simulink model "Copy_of_Controller"  (R2018b)
settings: configuration reference "control_config" (kept outside this file)
values from neighbouring files (symbols this model uses):
  CONTROL_EXPORT = Simulink.Parameter(CONTROL_EXPORT_VALUE)    [controller_model_init.m]
  CONTROL_PARAM = Simulink.Parameter(CONTROL_PARAM_VALUE)    [controller_model_init.m]
undefined symbols (not defined in the file or in its folder): actuator_cmd, CONTROL_CONST, ControlMode, DiscIntNeverNeededParam, phi_cmd, theta_cmd, timestamp, w_cmd
libraries: simulink x34, FMT_Model_Lib x19
(part 1 of 4)
settings Model: Creator=jc  LastModifiedBy=zouji
settings ConfigSetRef: SourceLocation=Base Workspace

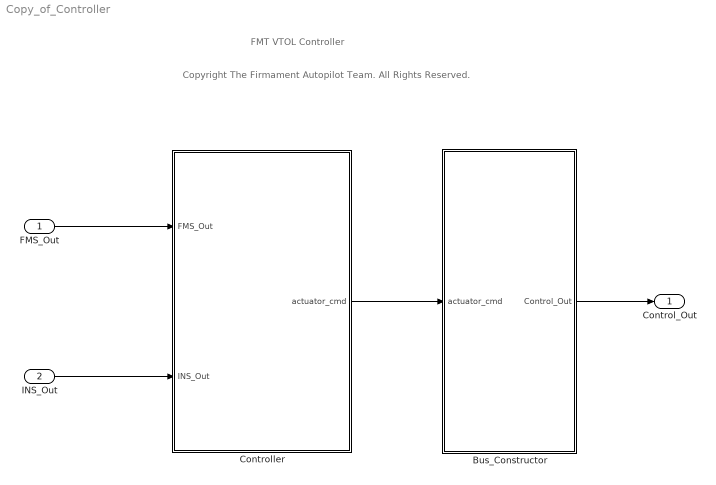
== system Copy_of_Controller ==
  note: Copyright The Firmament Autopilot Team. All Rights Reserved.
  note: FMT VTOL Controller
  FMS_Out : Inport  OutDataTypeStr=Bus: FMS_Out_Bus
  INS_Out : Inport  Port=2  OutDataTypeStr=Bus: INS_Out_Bus
  Bus_Constructor : Subsystem
  Controller : Subsystem
  Control_Out : Outport  OutDataTypeStr=Bus: Control_Out_Bus
  wires:
  FMS_Out/1 -> Controller/1(FMS_Out)
  INS_Out/1 -> Controller/2(INS_Out)
  Controller/1(actuator_cmd) -> Bus_Constructor/1(actuator_cmd)
  Bus_Constructor/1(Control_Out) -> Control_Out/1

== system Copy_of_Controller/Bus_Constructor ==
  actuator_cmd : Inport
  Bus Assignment : BusAssignment  AssignedSignals=actuator_cmd,timestamp
  Constant : Constant  Value=0  OutDataTypeStr=Bus: Control_Out_Bus
  timestamp : Subsystem  mask{sample_time=CONTROL_EXPORT.period}
      mask prompts: sample_time "sample time (ms)"
  Control_Out : Outport
  wires:
  actuator_cmd/1 -> Bus Assignment/2
  Constant/1 -> Bus Assignment/1
  Bus Assignment/1 -> Control_Out/1
  timestamp/1(timestamp_ms) -> Bus Assignment/3

== system Copy_of_Controller/Controller ==
  FMS_Out : Inport
  INS_Out : Inport  Port=2
  FW_Controller : Subsystem  TreatAsAtomicUnit=on
  MC_Controller : Subsystem  TreatAsAtomicUnit=on
  Merge : Merge
  VTOL_Control_Allocation : Subsystem
  switch-case : Subsystem
  actuator_cmd : Outport
  wires:
  INS_Out/1 -> MC_Controller/2(INS_Out), FW_Controller/2(INS_Out)
  FW_Controller/1(VTOL_actuator_cmd) -> Merge/1
  switch-case/1(FW_Trigger) -> FW_Controller/Action
  switch-case/2(MC_Trigger) -> MC_Controller/Action
  FMS_Out/1 -> MC_Controller/1(FMS_Out), FW_Controller/1(FMS_Out), VTOL_Control_Allocation/1(FMS_Out), switch-case/1(FMS_Out)
  MC_Controller/1(VTOL_actuator_cmd) -> Merge/2
  Merge/1 -> VTOL_Control_Allocation/2(VTOL_actuator_cmd)
  VTOL_Control_Allocation/1(actuator_cmd) -> actuator_cmd/1

== system Copy_of_Controller/Bus_Constructor/timestamp ==
  Constant : Constant  Value=sample_time
  Data Type Conversion : DataTypeConversion  OutDataTypeStr=uint32
  Discrete-Time Integrator : DiscreteIntegrator  IntegratorMethod=Accumulation: Forward Euler  SampleTime=-1  ICPrevOutput=DiscIntNeverNeededParam  ICPrevScaledInput=DiscIntNeverNeededParam
  timestamp_ms : Outport
  wires:
  Discrete-Time Integrator/1 -> Data Type Conversion/1
  Constant/1 -> Discrete-Time Integrator/1
  Data Type Conversion/1 -> timestamp_ms/1

== system Copy_of_Controller/Controller/FW_Controller ==
  FMS_Out : Inport
  INS_Out : Inport  Port=2
  Action Port : ActionPort  InitializeStates=reset  ActionType=case
  Aux_MC_Controller : Subsystem
  Effective_Factor : Subsystem
  FW_Controller : Subsystem
  Signal_Select : Subsystem
  VTOL_actuator_cmd : Outport  VectorParamsAs1DForOutWhenUnconnected=on
  wires:
  INS_Out/1 -> Aux_MC_Controller/3(INS_Out), FW_Controller/2(INS_Out), Effective_Factor/2(INS_Out)
  FW_Controller/3(aux_mc_cmd) -> Aux_MC_Controller/2(aux_cmd)
  FMS_Out/1 -> Aux_MC_Controller/1(FMS_Out), Signal_Select/1(FMS_Out), FW_Controller/1(FMS_Out), Effective_Factor/1(FMS_Out)
  Effective_Factor/2(factor_fw) -> FW_Controller/4(factor_fw)  "factor_fw"
  Effective_Factor/3(factor_mc) -> Aux_MC_Controller/4(factor_mc)  "factor_mc"
  Effective_Factor/1(VT) -> FW_Controller/3(VT)
  FW_Controller/1(fw_torque_cmd) -> Signal_Select/2(fw_torque_cmd)  "fw_torque_cmd"
  FW_Controller/2(fw_force_cmd) -> Signal_Select/3(fw_force_cmd)  "fw_force_cmd"
  Aux_MC_Controller/1(mc_torque_cmd) -> Signal_Select/4(mc_torque_cmd)  "aux_torque_cmd"
  Aux_MC_Controller/2(mc_force_cmd) -> Signal_Select/5(mc_force_cmd)  "aux_force_cmd"
  Signal_Select/1(VTOL_actuator_cmd) -> VTOL_actuator_cmd/1

== system Copy_of_Controller/Controller/MC_Controller ==
  FMS_Out : Inport
  INS_Out : Inport  Port=2
  Action Port : ActionPort  InitializeStates=reset  ActionType=default
  Bus Creator : BusCreator  Inputs=4
  Constant : Constant  Value=[0;0;0]  VectorParams1D=off  OutDataTypeStr=single
  Constant1 : Constant  Value=[0;0;0]  VectorParams1D=off  OutDataTypeStr=single
  Horizontal_Control : Subsystem
  Vertical_Control : Subsystem
  VTOL_actuator_cmd : Outport
  wires:
  Bus Creator/1 -> VTOL_actuator_cmd/1
  Horizontal_Control/1(torque_cmd_B) -> Bus Creator/3  "mc_torque_cmd"
  INS_Out/1 -> Vertical_Control/2(INS_Out), Horizontal_Control/2(INS_Out)
  Vertical_Control/1(force_cmd_B) -> Bus Creator/4  "mc_force_cmd"
  FMS_Out/1 -> Vertical_Control/1(FMS_Out), Horizontal_Control/1(FMS_Out)
  Constant/1 -> Bus Creator/1  "fw_torque_cmd"
  Constant1/1 -> Bus Creator/2  "fw_force_cmd"

== system Copy_of_Controller/Controller/VTOL_Control_Allocation ==
  FMS_Out : Inport
  VTOL_actuator_cmd : Inport  Port=2
  Bus Selector : BusSelector  OutputSignals=mc_torque_cmd,mc_force_cmd,fw_torque_cmd,fw_force_cmd
  Bus_Construct : Subsystem
  VTOL_Control_Allocation : Subsystem  Variant=on
      settings: GeneratePreprocessorConditionals=on
  actuator_cmd : Outport  VectorParamsAs1DForOutWhenUnconnected=on
  wires:
  FMS_Out/1 -> VTOL_Control_Allocation/1(FMS_Out)
  Bus_Construct/1(actuator_cmd) -> actuator_cmd/1
  VTOL_Control_Allocation/1(actuator_cmd) -> Bus_Construct/1(vtol_actuator_cmd)
  VTOL_actuator_cmd/1 -> Bus Selector/1
  Bus Selector/1 -> VTOL_Control_Allocation/2(mc_torque_cmd)  "<mc_torque_cmd>"
  Bus Selector/2 -> VTOL_Control_Allocation/3(mc_force_cmd)  "<mc_force_cmd>"
  Bus Selector/3 -> VTOL_Control_Allocation/4(fw_torque_cmd)  "<fw_torque_cmd>"
  Bus Selector/4 -> VTOL_Control_Allocation/5(fw_force_cmd)  "<fw_force_cmd>"

== system Copy_of_Controller/Controller/switch-case ==
  FMS_Out : Inport
  Bus Selector : BusSelector  OutputSignals=ext_state
  Data Type Conversion : DataTypeConversion  OutDataTypeStr=Enum: VTOLState
  Switch Case1 : SwitchCase  CaseConditions={[VTOLState.Fixwing, VTOLState.ForwardTrans, VTOLState.BackwardTrans, VTOLState.Stall]}
  FW_Trigger : Outport  VectorParamsAs1DForOutWhenUnconnected=on
  MC_Trigger : Outport  Port=2  VectorParamsAs1DForOutWhenUnconnected=on
  wires:
  Data Type Conversion/1 -> Switch Case1/1
  FMS_Out/1 -> Bus Selector/1
  Bus Selector/1 -> Data Type Conversion/1  "<ext_state>"
  Switch Case1/2 -> MC_Trigger/1
  Switch Case1/1 -> FW_Trigger/1

== system Copy_of_Controller/Controller/FW_Controller/Aux_MC_Controller ==
  FMS_Out : Inport
  aux_cmd : Inport  Port=2
  INS_Out : Inport  Port=3
  factor_mc : Inport  Port=4
  Attitude_Controller : Subsystem
  Aux_Commander : Subsystem
  Saturation1 : Saturate  UpperLimit=1  LowerLimit=-1
  Saturation2 : Saturate  UpperLimit=1  LowerLimit=-1
  Vertical_Control : Subsystem
  mc_torque_cmd : Outport
  mc_force_cmd : Outport  Port=2  VectorParamsAs1DForOutWhenUnconnected=on
  wires:
  INS_Out/1 -> Attitude_Controller/2(INS_Out), Vertical_Control/3(INS_Out)
  aux_cmd/1 -> Aux_Commander/1(aux_cmd)
  FMS_Out/1 -> Aux_Commander/2(FMS_Out)
  Aux_Commander/1(Aux_FMS_Out) -> Attitude_Controller/1(FMS_Out), Vertical_Control/2(FMS_Out)
  Attitude_Controller/1(rate_dot_cmd_B) -> Saturation2/1
  Saturation2/1 -> mc_torque_cmd/1
  Vertical_Control/1(force_cmd_B) -> Saturation1/1
  Saturation1/1 -> mc_force_cmd/1
  factor_mc/1 -> Vertical_Control/1(factor_mc), Attitude_Controller/3(factor_mc)

== system Copy_of_Controller/Controller/FW_Controller/Effective_Factor ==
  FMS_Out : Inport
  INS_Out : Inport  Port=2
  Bus Selector : BusSelector  OutputSignals=ext_state
  Constant : Constant  Value=0  OutDataTypeStr=single
  Constant1 : Constant  OutDataTypeStr=single
  Constant2 : Constant  OutDataTypeStr=single
  Constant6 : Constant  Value=0  OutDataTypeStr=single
  Demux : Demux  Outputs=2
  First Order LPF1 : FMT_Model_Lib/Filter/First Order LPF  fc=1
      settings: SourceProductName=FMT Toolbox
  First Order LPF3 : FMT_Model_Lib/Filter/First Order LPF  fc=0.5
      settings: SourceProductName=FMT Toolbox
  Fly_Speed : Subsystem
  Multiport Switch : MultiPortSwitch  DataPortOrder=Zero-based contiguous  Inputs=5  zeroidx=on
  Mux : Mux  Inputs=2
  Mux2 : Mux  Inputs=2
  VT : Outport  VectorParamsAs1DForOutWhenUnconnected=on
  factor_fw : Outport  Port=2  VectorParamsAs1DForOutWhenUnconnected=on
  factor_mc : Outport  Port=3  VectorParamsAs1DForOutWhenUnconnected=on
  wires:
  INS_Out/1 -> Fly_Speed/1(INS_Out)
  Fly_Speed/1(VT) -> VT/1  "VT"
  FMS_Out/1 -> Bus Selector/1
  Bus Selector/1 -> Multiport Switch/1  "<ext_state>"
  Constant/1 -> Mux/1
  Constant1/1 -> Mux/2
  First Order LPF1/1 -> factor_fw/1
  First Order LPF3/1 -> factor_mc/1
  Mux/1 -> Multiport Switch/2, Multiport Switch/3, Multiport Switch/5, Multiport Switch/6
  Mux2/1 -> Multiport Switch/4
  Constant2/1 -> Mux2/1
  Constant6/1 -> Mux2/2
  Multiport Switch/1 -> Demux/1
  Demux/2 -> First Order LPF3/1
  Demux/1 -> First Order LPF1/1

== system Copy_of_Controller/Controller/FW_Controller/FW_Controller ==
  FMS_Out : Inport
  INS_Out : Inport  Port=2
  VT : Inport  Port=3
  factor_fw : Inport  Port=4
  Attitude_Control : Subsystem
  Lateral_Control : Subsystem
  Mux : Mux  Inputs=2
  Saturation1 : Saturate  UpperLimit=1  LowerLimit=-1
  Selector : Selector  InputPortWidth=3  IndexOptions=Index vector (dialog)  Indices=1  OutputSizes=1
  TECS_Core : Subsystem
  Throttle_Command : Subsystem
  fw_torque_cmd : Outport  VectorParamsAs1DForOutWhenUnconnected=on
  fw_force_cmd : Outport  Port=2  VectorParamsAs1DForOutWhenUnconnected=on
  aux_mc_cmd : Outport  Port=3  VectorParamsAs1DForOutWhenUnconnected=on
  wires:
  INS_Out/1 -> TECS_Core/1(INS_Out), Lateral_Control/2(INS_Out), Attitude_Control/4(INS_Out)
  Lateral_Control/1(phi_cmd) -> Mux/1  "fw_phi_cmd"
  Mux/1 -> Attitude_Control/5(att_cmd)
  TECS_Core/1(theta_cmd) -> Mux/2  "fw_theta_cmd"
  FMS_Out/1 -> TECS_Core/2(FMS_Out), Throttle_Command/2(FMS_Out), Lateral_Control/1(FMS_Out), Attitude_Control/2(FMS_Out)
  Attitude_Control/1(ang_acc_cmd) -> Saturation1/1
  Saturation1/1 -> fw_torque_cmd/1
  VT/1 -> Attitude_Control/3(VT), TECS_Core/3(VT)
  Attitude_Control/2(aux_mc_cmd) -> Selector/1, aux_mc_cmd/1  "aux_mc_cmd"
  TECS_Core/2(throttle_cmd) -> Throttle_Command/1(fw_throttle_cmd)  "fw_throttle_cmd"
  Throttle_Command/1(fw_force_cmd) -> fw_force_cmd/1
  Selector/1 -> TECS_Core/4(fw_phi_sp)
  factor_fw/1 -> Attitude_Control/1(factor_fw)

== system Copy_of_Controller/Controller/FW_Controller/Signal_Select ==
  FMS_Out : Inport
  fw_torque_cmd : Inport  Port=2
  fw_force_cmd : Inport  Port=3
  mc_torque_cmd : Inport  Port=4
  mc_force_cmd : Inport  Port=5
  Bus Creator : BusCreator  Inputs=4
  Bus Selector1 : BusSelector  OutputSignals=ctrl_mode
  Manual : simulink/Logic and Bit Operations/Compare To Constant  relop===  const=uint8(ControlMode.Manual)  OutDataTypeStr=boolean
  Manual_Command : Subsystem
  Switch : Switch  Criteria=u2 > Threshold
  VTOL_actuator_cmd : Outport
  wires:
  mc_force_cmd/1 -> Bus Creator/4  "mc_force_cmd"
  fw_torque_cmd/1 -> Bus Creator/1  "fw_torque_cmd"
  fw_force_cmd/1 -> Bus Creator/2  "fw_force_cmd"
  mc_torque_cmd/1 -> Bus Creator/3  "mc_torque_cmd"
  Bus Selector1/1 -> Manual/1  "<ctrl_mode>"
  FMS_Out/1 -> Manual_Command/1(FMS_Out), Bus Selector1/1
  Manual/1 -> Switch/2
  Bus Creator/1 -> Switch/3
  Switch/1 -> VTOL_actuator_cmd/1
  Manual_Command/1(vtol_actuator_cmd) -> Switch/1

== system Copy_of_Controller/Controller/MC_Controller/Horizontal_Control ==
  FMS_Out : Inport
  INS_Out : Inport  Port=2
  Attitude_Controller : Subsystem
  Velocity_Controller : Subsystem
  torque_cmd_B : Outport
  wires:
  Attitude_Controller/1(rate_dot_cmd_B) -> torque_cmd_B/1
  FMS_Out/1 -> Attitude_Controller/2(FMS_Out), Velocity_Controller/1(FMS_Out)
  INS_Out/1 -> Velocity_Controller/2(INS_Out), Attitude_Controller/3(INS_Out)
  Velocity_Controller/1(att_cmd_B_rad) -> Attitude_Controller/1(att_cmd_B_rad)

== system Copy_of_Controller/Controller/MC_Controller/Vertical_Control ==
  FMS_Out : Inport
  INS_Out : Inport  Port=2
  Signal_Select : Subsystem
  Veloxity_Z_Controller : Subsystem
  force_cmd_B : Outport
  wires:
  INS_Out/1 -> Veloxity_Z_Controller/2(INS_Out)
  FMS_Out/1 -> Signal_Select/1(FMS_Out), Veloxity_Z_Controller/1(FMS_Out)
  Veloxity_Z_Controller/1(throttle_cmd) -> Signal_Select/2(throttle_cmd)
  Signal_Select/1(force_cmd) -> force_cmd_B/1

== system Copy_of_Controller/Controller/VTOL_Control_Allocation/Bus_Construct ==
  vtol_actuator_cmd : Inport
  Constant : Constant  Value=zeros(7,1)  VectorParams1D=off  OutDataTypeStr=uint16
  Mux : Mux  Inputs=2
  Reshape : Reshape  OutputDimensionality=Column vector (2-D)  OutputDimensions=[16,1]
  actuator_cmd : Outport  VectorParamsAs1DForOutWhenUnconnected=on
  wires:
  Reshape/1 -> actuator_cmd/1
  Constant/1 -> Mux/2
  Mux/1 -> Reshape/1
  vtol_actuator_cmd/1 -> Mux/1

== system Copy_of_Controller/Controller/VTOL_Control_Allocation/VTOL_Control_Allocation ==
  note: 1) Add Subsystem or Model blocks as valid variant choices.
      | 2) You cannot connect blocks at this level. At simulation, connectivity is automatically
      | determined, based on the active variant and port name matching.
  FMS_Out : Inport
  mc_torque_cmd : Inport  Port=2
  mc_force_cmd : Inport  Port=3
  fw_torque_cmd : Inport  Port=4
  fw_force_cmd : Inport  Port=5
  VTOL1 : Subsystem  TreatAsAtomicUnit=on  VariantControl=AIRFRAME==1
      mask Display: image('.\figures\vtol_1.png');
  VTOL2 : Subsystem  TreatAsAtomicUnit=on  VariantControl=AIRFRAME==2
      mask Display: image('.\figures\vtol_2.png');
  actuator_cmd : Outport

== system Copy_of_Controller/Controller/FW_Controller/Aux_MC_Controller/Attitude_Controller ==
  FMS_Out : Inport
  INS_Out : Inport  Port=2
  factor_mc : Inport  Port=3
  Bus Selector : BusSelector  OutputSignals=phi_cmd,theta_cmd
  Inner_Loop : Subsystem
  Mux : Mux  Inputs=2
  Outter_Loop : Subsystem
  rate_dot_cmd_B : Outport
  wires:
  INS_Out/1 -> Inner_Loop/2(INS_Out), Outter_Loop/2(INS_Out)
  FMS_Out/1 -> Bus Selector/1, Inner_Loop/3(FMS_Out)
  Mux/1 -> Outter_Loop/1(att_cmd_rad)
  Outter_Loop/1(euler_rate_cmd_radPs) -> Inner_Loop/1(euler_rate_cmd_radPs)
  Inner_Loop/1(rate_dot_cmd_B) -> rate_dot_cmd_B/1
  Bus Selector/1 -> Mux/1  "<phi_cmd>"
  Bus Selector/2 -> Mux/2  "<theta_cmd>"
  factor_mc/1 -> Inner_Loop/4(factor_mc)

== system Copy_of_Controller/Controller/FW_Controller/Aux_MC_Controller/Aux_Commander ==
  aux_cmd : Inport
  FMS_Out : Inport  Port=2
  Bus Assignment : BusAssignment  AssignedSignals=phi_cmd,theta_cmd,w_cmd
  Commander : Subsystem  Commented=on
  Demux : Demux  Outputs=3
  Aux_FMS_Out : Outport  VectorParamsAs1DForOutWhenUnconnected=on
  wires:
  aux_cmd/1 -> Demux/1
  Demux/1 -> Bus Assignment/2
  Demux/2 -> Bus Assignment/3
  Demux/3 -> Bus Assignment/4
  FMS_Out/1 -> Bus Assignment/1
  Bus Assignment/1 -> Aux_FMS_Out/1

== system Copy_of_Controller/Controller/FW_Controller/Aux_MC_Controller/Vertical_Control ==
  factor_mc : Inport
  FMS_Out : Inport  Port=2
  INS_Out : Inport  Port=3
  Constant : Constant  Value=0  OutDataTypeStr=single
  Mux : Mux  Inputs=3
  Veloxity_Z_Controller : Subsystem
  force_cmd_B : Outport
  wires:
  INS_Out/1 -> Veloxity_Z_Controller/3(INS_Out)
  FMS_Out/1 -> Veloxity_Z_Controller/2(FMS_Out)
  factor_mc/1 -> Veloxity_Z_Controller/1(factor_mc)
  Mux/1 -> force_cmd_B/1
  Veloxity_Z_Controller/1(throttle_cmd) -> Mux/3
  Constant/1 -> Mux/2, Mux/1

== system Copy_of_Controller/Controller/FW_Controller/Effective_Factor/Fly_Speed ==
  note: If airspeed invalid or small, use ground speed
  INS_Out : Inport
  Add : Sum
  Bus Selector1 : BusSelector  OutputSignals=vn,ve
  Bus Selector2 : BusSelector  OutputSignals=flag
  Bus Selector3 : BusSelector  OutputSignals=airspeed
  Compare To Zero : simulink/Logic and Bit Operations/Compare To Zero  relop===  OutDataTypeStr=boolean
  First Order LPF3 : FMT_Model_Lib/Filter/First Order LPF  fc=10
      settings: SourceProductName=FMT Toolbox
  Fly_Direction : Subsystem
  Logical Operator : Logic  AllPortsSameDT=off  OutDataTypeStr=boolean
  Logical Operator1 : Logic  Operator=OR  AllPortsSameDT=off  OutDataTypeStr=boolean
  Multiply : Product
  Relay : Relay  OnSwitchValue=10  OffSwitchValue=6
  Saturation1 : Saturate  UpperLimit=100  LowerLimit=0.1
  Sqrt : Sqrt  SaturateOnIntegerOverflow=on
  Square2 : Math  Operator=square  SaturateOnIntegerOverflow=on
  Square3 : Math  Operator=square  SaturateOnIntegerOverflow=on
  Switch : Switch  Criteria=u2 > Threshold
  airspeed_valid : simulink/Logic and Bit Operations/Bitwise Operator  logicop=AND  UseBitMask=on  BitMask=bin2dec('1000000000')  BitMaskRealWorld=Stored Integer
  vel_valid : simulink/Logic and Bit Operations/Bitwise Operator  logicop=AND  UseBitMask=on  BitMask=bin2dec('10000')  BitMaskRealWorld=Stored Integer
  VT : Outport
  wires:
  INS_Out/1 -> Bus Selector1/1, Fly_Direction/1(INS_Out), Bus Selector3/1, Bus Selector2/1
  Bus Selector3/1 -> Relay/1, Switch/1  "<airspeed>"
  Bus Selector1/2 -> Square3/1  "<ve>"
  Bus Selector1/1 -> Square2/1  "<vn>"
  Bus Selector2/1 -> vel_valid/1, airspeed_valid/1  "<flag>"
  Square3/1 -> Add/2
  Add/1 -> Sqrt/1
  Square2/1 -> Add/1
  Fly_Direction/1(sign) -> Multiply/1
  Multiply/1 -> Switch/3
  Sqrt/1 -> Multiply/2
  First Order LPF3/1 -> VT/1
  Saturation1/1 -> First Order LPF3/1
  airspeed_valid/1 -> Logical Operator/2
  Switch/1 -> Saturation1/1
  Relay/1 -> Logical Operator/1
  vel_valid/1 -> Compare To Zero/1
  Logical Operator1/1 -> Switch/2
  Logical Operator/1 -> Logical Operator1/1
  Compare To Zero/1 -> Logical Operator1/2

== system Copy_of_Controller/Controller/FW_Controller/FW_Controller/Attitude_Control ==
  factor_fw : Inport
  FMS_Out : Inport  Port=2
  VT : Inport  Port=3
  INS_Out : Inport  Port=4
  att_cmd : Inport  Port=5
  Bus Selector : BusSelector  OutputSignals=w_cmd
  Innerloop_Rate_Control : Subsystem
  Mux : Mux  Inputs=2
  Outloop_Angle_Control : Subsystem
  ang_acc_cmd : Outport
  aux_mc_cmd : Outport  Port=2
  wires:
  INS_Out/1 -> Innerloop_Rate_Control/3(INS_Out), Outloop_Angle_Control/3(INS_Out)
  FMS_Out/1 -> Bus Selector/1, Innerloop_Rate_Control/2(FMS_Out), Outloop_Angle_Control/4(FMS_Out)
  Outloop_Angle_Control/2(fw_euler_rate_cmd) -> Innerloop_Rate_Control/1(fw_euler_rate_cmd)
  Innerloop_Rate_Control/1(rate_dot_cmd) -> ang_acc_cmd/1
  att_cmd/1 -> Outloop_Angle_Control/1(att_cmd)
  VT/1 -> Innerloop_Rate_Control/4(VT), Outloop_Angle_Control/2(VT)
  Outloop_Angle_Control/1(fw_att_cmd) -> Mux/1
  Bus Selector/1 -> Mux/2  "<w_cmd>"
  Mux/1 -> aux_mc_cmd/1
  factor_fw/1 -> Innerloop_Rate_Control/5(factor_fw)

== system Copy_of_Controller/Controller/FW_Controller/FW_Controller/Lateral_Control ==
  FMS_Out : Inport
  INS_Out : Inport  Port=2
  Atan : Trigonometry  Operator=atan
  Bus Selector : BusSelector  OutputSignals=ay_cmd
  Saturation : Saturate  UpperLimit=CONTROL_PARAM.FW_ROLL_PITCH_CMD_LIM  LowerLimit=-CONTROL_PARAM.FW_ROLL_PITCH_CMD_LIM
  Terminator : Terminator
  g_force : Gain  Gain=1/9.81
  phi_cmd : Outport
  wires:
  FMS_Out/1 -> Bus Selector/1
  Bus Selector/1 -> g_force/1  "<ay_cmd>"
  g_force/1 -> Atan/1
  Atan/1 -> Saturation/1  "phi_cmd"
  INS_Out/1 -> Terminator/1
  Saturation/1 -> phi_cmd/1

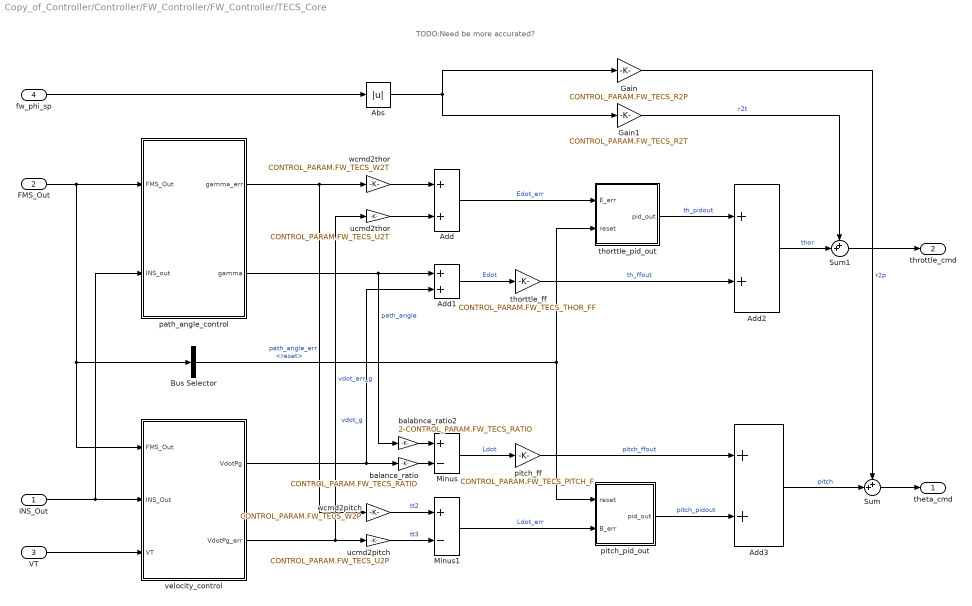
== system Copy_of_Controller/Controller/FW_Controller/FW_Controller/TECS_Core ==
  note: TODO:Need be more accurated?
  INS_Out : Inport
  FMS_Out : Inport  Port=2
  VT : Inport  Port=3
  fw_phi_sp : Inport  Port=4
  Abs : Abs
  Add{,1..3} (4 alike) : Sum
  Bus Selector : BusSelector  OutputSignals=reset
  Gain : Gain  Gain=CONTROL_PARAM.FW_TECS_R2P
  Gain1 : Gain  Gain=CONTROL_PARAM.FW_TECS_R2T
  Minus : Sum  Inputs=+-
  Minus1 : Sum  Inputs=+-
  Sum : Sum  Inputs=++|
  Sum1 : Sum  Inputs=++|
  balabnce_ratio2 : Gain  Gain=2-CONTROL_PARAM.FW_TECS_RATIO
  balance_ratio : Gain  Gain=CONTROL_PARAM.FW_TECS_RATIO
  path_angle_control : Subsystem
  pitch_ff : Gain  Gain=CONTROL_PARAM.FW_TECS_PITCH_F
  pitch_pid_out : Subsystem
  thorttle_ff : Gain  Gain=CONTROL_PARAM.FW_TECS_THOR_FF
  thorttle_pid_out : Subsystem
  ucmd2pitch : Gain  Gain=CONTROL_PARAM.FW_TECS_U2P
  ucmd2thor : Gain  Gain=CONTROL_PARAM.FW_TECS_U2T
  velocity_control : Subsystem
  wcmd2pitch : Gain  Gain=CONTROL_PARAM.FW_TECS_W2P
  wcmd2thor : Gain  Gain=CONTROL_PARAM.FW_TECS_W2T
  theta_cmd : Outport
  throttle_cmd : Outport  Port=2
  wires:
  INS_Out/1 -> path_angle_control/2(INS_out), velocity_control/2(INS_Out)
  path_angle_control/1(gamma_err) -> wcmd2pitch/1, wcmd2thor/1  "path_angle_err"
  velocity_control/2(VdotPg_err) -> ucmd2thor/1, ucmd2pitch/1  "vdot_err_g"
  velocity_control/1(VdotPg) -> Add1/2, balance_ratio/1  "vdot_g"
  path_angle_control/2(gamma) -> balabnce_ratio2/1, Add1/1  "path_angle"
  Minus/1 -> pitch_ff/1  "Ldot"
  Add1/1 -> thorttle_ff/1  "Edot"
  thorttle_ff/1 -> Add2/2  "th_ffout"
  Bus Selector/1 -> pitch_pid_out/1(reset), thorttle_pid_out/2(reset)  "<reset>"
  pitch_ff/1 -> Add3/1  "pitch_ffout"
  Add/1 -> thorttle_pid_out/1(E_err)  "Edot_err"
  thorttle_pid_out/1(pid_out) -> Add2/1  "th_pidout"
  Minus1/1 -> pitch_pid_out/2(B_err)  "Ldot_err"
  pitch_pid_out/1(pid_out) -> Add3/2  "pitch_pidout"
  balabnce_ratio2/1 -> Minus/1
  wcmd2thor/1 -> Add/1
  ucmd2thor/1 -> Add/2
  FMS_Out/1 -> Bus Selector/1, velocity_control/1(FMS_Out), path_angle_control/1(FMS_Out)
  Sum/1 -> theta_cmd/1
  Sum1/1 -> throttle_cmd/1
  Add2/1 -> Sum1/2  "thor"
  Gain1/1 -> Sum1/1  "r2t"
  fw_phi_sp/1 -> Abs/1
  wcmd2pitch/1 -> Minus1/1  "tt2"
  ucmd2pitch/1 -> Minus1/2  "tt3"
  Gain/1 -> Sum/1  "r2p"
  Add3/1 -> Sum/2  "pitch"
  Abs/1 -> Gain/1, Gain1/1
  balance_ratio/1 -> Minus/2
  VT/1 -> velocity_control/3(VT)

== system Copy_of_Controller/Controller/FW_Controller/FW_Controller/Throttle_Command ==
  fw_throttle_cmd : Inport
  FMS_Out : Inport  Port=2
  Bias : Bias  Bias=-1
  Bus Selector : BusSelector  OutputSignals=ctrl_mode
  Bus Selector1 : BusSelector  OutputSignals=throttle_cmd
  Compare To Constant : simulink/Logic and Bit Operations/Compare To Constant  relop=<=  const=uint8(ControlMode.Stabilize)  OutDataTypeStr=boolean
  Constant : Constant  Value=0  OutDataTypeStr=single
  Gain : Gain  Gain=1/1000  OutDataTypeStr=single
  Mux1 : Mux  Inputs=3
  Saturation : Saturate  UpperLimit=1  LowerLimit=-1
  Saturation2 : Saturate  UpperLimit=1  LowerLimit=-1
  Sum : Sum  Inputs=|++
  Switch : Switch  Criteria=u2 > Threshold
  cruise_throttle : Constant  Value=CONTROL_PARAM.FW_CRUISE_THRO  OutDataTypeStr=Inherit: Inherit via back propagation
  fw_force_cmd : Outport
  wires:
  Saturation2/1 -> fw_force_cmd/1
  Constant/1 -> Mux1/3, Mux1/2
  fw_throttle_cmd/1 -> Saturation/1, Sum/1
  Mux1/1 -> Saturation2/1
  cruise_throttle/1 -> Sum/2
  Saturation/1 -> Switch/3
  Compare To Constant/1 -> Switch/2
  FMS_Out/1 -> Bus Selector1/1, Bus Selector/1
  Bus Selector/1 -> Compare To Constant/1  "<ctrl_mode>"
  Bus Selector1/1 -> Gain/1  "<throttle_cmd>"
  Gain/1 -> Bias/1
  Switch/1 -> Mux1/1
  Bias/1 -> Switch/1

== system Copy_of_Controller/Controller/FW_Controller/Signal_Select/Manual_Command ==
  FMS_Out : Inport
  Bus Creator1 : BusCreator  Inputs=4
  Bus Selector1 : BusSelector  OutputSignals=u_cmd
  Bus Selector2 : BusSelector  OutputSignals=p_cmd,q_cmd,r_cmd
  Constant : Constant  Value=[0 0 0]  OutDataTypeStr=single
  Constant1 : Constant  Value=[0 0 0]  OutDataTypeStr=single
  Constant2 : Constant  Value=0  OutDataTypeStr=single
  Mux : Mux  Inputs=3
  Mux1 : Mux  Inputs=3
  vtol_actuator_cmd : Outport
  wires:
  Mux1/1 -> Bus Creator1/2  "fw_force_cmd"
  Mux/1 -> Bus Creator1/1  "fw_torque_cmd"
  Constant2/1 -> Mux1/3, Mux1/2
  Bus Selector2/2 -> Mux/2  "<q_cmd>"
  Constant1/1 -> Bus Creator1/4  "mc_force_cmd"
  Bus Selector2/1 -> Mux/1  "<p_cmd>"
  Constant/1 -> Bus Creator1/3  "mc_torque_cmd"
  Bus Selector2/3 -> Mux/3  "<r_cmd>"
  Bus Creator1/1 -> vtol_actuator_cmd/1
  FMS_Out/1 -> Bus Selector2/1, Bus Selector1/1
  Bus Selector1/1 -> Mux1/1  "<u_cmd>"

== system Copy_of_Controller/Controller/MC_Controller/Horizontal_Control/Attitude_Controller ==
  att_cmd_B_rad : Inport
  FMS_Out : Inport  Port=2
  INS_Out : Inport  Port=3
  Inner_Loop : Subsystem
  Outter_Loop : Subsystem
  rate_dot_cmd_B : Outport
  wires:
  INS_Out/1 -> Inner_Loop/2(INS_Out), Outter_Loop/2(INS_Out)
  FMS_Out/1 -> Inner_Loop/3(FMS_Out), Outter_Loop/3(FMS_Out)
  att_cmd_B_rad/1 -> Outter_Loop/1(att_cmd_rad)
  Outter_Loop/1(euler_rate_cmd_radPs) -> Inner_Loop/1(euler_rate_cmd_radPs)
  Inner_Loop/1(rate_dot_cmd_B) -> rate_dot_cmd_B/1

== system Copy_of_Controller/Controller/MC_Controller/Horizontal_Control/Velocity_Controller ==
  FMS_Out : Inport
  INS_Out : Inport  Port=2
  Accel_to_Attitude_CMD : Subsystem
  Bus Selector : BusSelector  OutputSignals=reset
  Error : Subsystem
  PID_Controller : Subsystem
  Signal_Select : Subsystem
  att_cmd_B_rad : Outport
  wires:
  FMS_Out/1 -> Signal_Select/2(FMS_Out), Error/2(FMS_Out), Bus Selector/1
  PID_Controller/1(accel_cmd_C) -> Signal_Select/1(acc_cmd_in)  "accel_cmd_C_mPs2"
  INS_Out/1 -> Error/1(INS_Out)
  Error/1(uv_err_C_mPs) -> PID_Controller/1(uv_err_C_mPs)
  Accel_to_Attitude_CMD/1(att_cmd_B_rad) -> att_cmd_B_rad/1
  Bus Selector/1 -> PID_Controller/2(reset)  "<reset>"
  Signal_Select/1(acc_cmd_out) -> Accel_to_Attitude_CMD/1(accel_cmd_C_mPs2)

== system Copy_of_Controller/Controller/MC_Controller/Vertical_Control/Signal_Select ==
  FMS_Out : Inport
  throttle_cmd : Inport  Port=2
  Bias : Bias  Bias=-1
  Bus Selector1 : BusSelector  OutputSignals=ctrl_mode
  Bus Selector2 : BusSelector  OutputSignals=throttle_cmd
  Compare To Constant : simulink/Logic and Bit Operations/Compare To Constant  relop=<=  const=uint8(ControlMode.Stabilize)  OutDataTypeStr=boolean
  Constant : Constant  Value=0  OutDataTypeStr=single
  Gain : Gain  Gain=1/1000  OutDataTypeStr=single
  Mux : Mux  Inputs=3
  Switch : Switch  Criteria=u2 > Threshold
  force_cmd : Outport
  wires:
  Bus Selector1/1 -> Compare To Constant/1  "<ctrl_mode>"
  Bus Selector2/1 -> Gain/1  "<throttle_cmd>"
  throttle_cmd/1 -> Switch/3
  Constant/1 -> Mux/2, Mux/1
  Compare To Constant/1 -> Switch/2
  Mux/1 -> force_cmd/1
  FMS_Out/1 -> Bus Selector1/1, Bus Selector2/1
  Switch/1 -> Mux/3
  Gain/1 -> Bias/1
  Bias/1 -> Switch/1

== system Copy_of_Controller/Controller/MC_Controller/Vertical_Control/Veloxity_Z_Controller ==
  FMS_Out : Inport
  INS_Out : Inport  Port=2
  Boosted_Throttle : Subsystem
  Bus Selector : BusSelector  OutputSignals=reset
  Error : Subsystem
  PID_Controller : Subsystem
  Sum : Sum  Inputs=|++
  hover_throttle : Constant  Value=CONTROL_PARAM.MC_HOVER_THRO  OutDataTypeStr=Inherit: Inherit via back propagation
  throttle_cmd : Outport
  wires:
  FMS_Out/1 -> Bus Selector/1, Error/1(FMS_Out)
  INS_Out/1 -> Error/2(INS_Out), Boosted_Throttle/2(INS_Out)
  Boosted_Throttle/1(boosted_thrust) -> Sum/1  "boosted_thrust"
  Error/1(vu_cmd_C_mPs) -> PID_Controller/1(vu_cmd_C_mPs)
  Bus Selector/1 -> PID_Controller/2(reset)  "<reset>"
  PID_Controller/1(thrust_cmd) -> Boosted_Throttle/1(thrust_cmd)
  hover_throttle/1 -> Sum/2
  Sum/1 -> throttle_cmd/1

== system Copy_of_Controller/Controller/VTOL_Control_Allocation/VTOL_Control_Allocation/VTOL1 ==
  FMS_Out : Inport
  mc_torque_cmd : Inport  Port=2
  mc_force_cmd : Inport  Port=3
  fw_torque_cmd : Inport  Port=4
  fw_force_cmd : Inport  Port=5
  Bus Selector : BusSelector  OutputSignals=status
  FW_Control_Allocation : Subsystem  mask{up_limit=CONTROL_PARAM.FW_OUT_MAX, lo_limit=CONTROL_PARAM.FW_OUT_MIN}
      mask prompts: up_limit "Upper Limit"; lo_limit "Lower Limit"
  MC_Control_Allocation : Subsystem  mask{up_lim=CONTROL_PARAM.MC_OUT_MAX, lo_lim=CONTROL_PARAM.MC_OUT_MIN}
      mask prompts: up_lim "Upper Limit"; lo_lim "Lower Limit"
  MC_Control_Allocation1 : Subsystem  Commented=on
  MC_Control_Allocation2 : Subsystem  Commented=on  mask{up_lim=CONTROL_PARAM.MC_OUT_MAX, lo_lim=CONTROL_PARAM.MC_OUT_MIN}
      mask prompts: up_lim "Upper Limit"; lo_lim "Lower Limit"
  Mux : Mux  Inputs=2
  Reshape : Reshape  OutputDimensionality=Column vector (2-D)  OutputDimensions=[16,1]
  actuator_cmd_routing : Subsystem
  actuator_cmd : Outport
  wires:
  actuator_cmd_routing/1(cmd_out) -> actuator_cmd/1
  Reshape/1 -> actuator_cmd_routing/1(cmd_in)
  mc_torque_cmd/1 -> MC_Control_Allocation/1(mc_torque_cmd)
  mc_force_cmd/1 -> MC_Control_Allocation/2(mc_force_cmd)
  fw_force_cmd/1 -> FW_Control_Allocation/2(fw_force_cmd)
  FMS_Out/1 -> FW_Control_Allocation/3(FMS_Out), Bus Selector/1
  fw_torque_cmd/1 -> FW_Control_Allocation/1(fw_torque_cmd)
  MC_Control_Allocation/1(mc_actuator_cmd) -> Mux/1
  FW_Control_Allocation/1(fw_actuator_cmd) -> Mux/2
  Mux/1 -> Reshape/1
  Bus Selector/1 -> actuator_cmd_routing/2(status)  "<status>"

== system Copy_of_Controller/Controller/VTOL_Control_Allocation/VTOL_Control_Allocation/VTOL2 ==
  FMS_Out : Inport
  mc_torque_cmd : Inport  Port=2
  mc_force_cmd : Inport  Port=3
  fw_torque_cmd : Inport  Port=4
  fw_force_cmd : Inport  Port=5
  Bus Selector : BusSelector  OutputSignals=status
  FW_Control_Allocation : Subsystem  mask{up_limit=CONTROL_PARAM.FW_OUT_MAX, lo_limit=CONTROL_PARAM.FW_OUT_MIN}
      mask prompts: up_limit "Upper Limit"; lo_limit "Lower Limit"
  MC_Control_Allocation : Subsystem  mask{up_lim=CONTROL_PARAM.MC_OUT_MAX, lo_lim=CONTROL_PARAM.MC_OUT_MIN}
      mask prompts: up_lim "Upper Limit"; lo_lim "Lower Limit"
  MC_Control_Allocation2 : Subsystem  Commented=on
  Mux : Mux  Inputs=2
  Reshape : Reshape  OutputDimensionality=Column vector (2-D)  OutputDimensions=[16,1]
  actuator_cmd_routing : Subsystem
  actuator_cmd : Outport
  wires:
  actuator_cmd_routing/1(cmd_out) -> actuator_cmd/1
  Reshape/1 -> actuator_cmd_routing/1(cmd_in)
  mc_torque_cmd/1 -> MC_Control_Allocation/1(mc_torque_cmd)
  mc_force_cmd/1 -> MC_Control_Allocation/2(mc_force_cmd)
  fw_force_cmd/1 -> FW_Control_Allocation/2(fw_force_cmd)
  FMS_Out/1 -> FW_Control_Allocation/3(FMS_Out), Bus Selector/1
  fw_torque_cmd/1 -> FW_Control_Allocation/1(fw_torque_cmd)
  MC_Control_Allocation/1(mc_actuator_cmd) -> Mux/1
  FW_Control_Allocation/1(fw_actuator_cmd) -> Mux/2
  Mux/1 -> Reshape/1
  Bus Selector/1 -> actuator_cmd_routing/2(status)  "<status>"

== system Copy_of_Controller/Controller/FW_Controller/Aux_MC_Controller/Attitude_Controller/Inner_Loop ==
  euler_rate_cmd_radPs : Inport
  INS_Out : Inport  Port=2
  FMS_Out : Inport  Port=3
  factor_mc : Inport  Port=4
  Bus Selector : BusSelector  OutputSignals=reset
  Rate_Controller : Subsystem
  Signal_Convert : Subsystem
  rate_dot_cmd_B : Outport
  wires:
  euler_rate_cmd_radPs/1 -> Signal_Convert/2(euler_rate_cmd)
  Signal_Convert/1(rate_cmd_radPs) -> Rate_Controller/1(rate_cmd_radPs)
  Rate_Controller/1(rate_dot_cmd_B) -> rate_dot_cmd_B/1
  INS_Out/1 -> Signal_Convert/3(INS_Out), Rate_Controller/2(INS_Out)
  FMS_Out/1 -> Bus Selector/1, Signal_Convert/1(FMS_Out)
  Bus Selector/1 -> Rate_Controller/3(reset)  "<reset>"
  factor_mc/1 -> Rate_Controller/4(factor_mc)

== system Copy_of_Controller/Controller/FW_Controller/Aux_MC_Controller/Attitude_Controller/Outter_Loop ==
  att_cmd_rad : Inport
  INS_Out : Inport  Port=2
  Attitude_Controller : Subsystem
  euler_rate_cmd_radPs : Outport
  wires:
  att_cmd_rad/1 -> Attitude_Controller/1(att_cmd_rad)
  INS_Out/1 -> Attitude_Controller/2(INS_Out)
  Attitude_Controller/1(euler_rate_cmd_radPs) -> euler_rate_cmd_radPs/1

== system Copy_of_Controller/Controller/FW_Controller/Aux_MC_Controller/Aux_Commander/Commander ==
  FMS_Out : Inport
  aux_cmd : Inport  Port=2
  Phi_Commander : Subsystem
  Theta_Commander : Subsystem
  W_Commander : Subsystem
  phi_cmd : Outport  VectorParamsAs1DForOutWhenUnconnected=on
  theta_cmd : Outport  Port=2  VectorParamsAs1DForOutWhenUnconnected=on
  w_cmd : Outport  Port=3  VectorParamsAs1DForOutWhenUnconnected=on
  wires:
  FMS_Out/1 -> W_Commander/1(FMS_Out), Theta_Commander/1(FMS_Out), Phi_Commander/1(FMS_Out)
  aux_cmd/1 -> Phi_Commander/2(aux_cmd), Theta_Commander/2(aux_cmd)
  Phi_Commander/1(phi_cmd) -> phi_cmd/1
  Theta_Commander/1(theta_cmd) -> theta_cmd/1
  W_Commander/1(w_cmd) -> w_cmd/1

== system Copy_of_Controller/Controller/FW_Controller/Aux_MC_Controller/Vertical_Control/Veloxity_Z_Controller ==
  note: Leave some margin
      | for att control
  factor_mc : Inport
  FMS_Out : Inport  Port=2
  INS_Out : Inport  Port=3
  Boosted_Throttle : Subsystem
  Bus Selector : BusSelector  OutputSignals=reset
  Error : Subsystem
  Logical Operator : Logic  Operator=OR  AllPortsSameDT=off  OutDataTypeStr=boolean
  Multiply : Product
  PID_Controller : Subsystem
  Relay : Relay  OnSwitchValue=0.3  OffSwitchValue=0.1  OnOutputValue=0  OffOutputValue=1
  Saturation : Saturate  UpperLimit=0.35  LowerLimit=-0.35
  Sum1 : Sum  Inputs=|++
  hover_throttle : Constant  Value=CONTROL_PARAM.MC_HOVER_THRO  OutDataTypeStr=Inherit: Inherit via back propagation
  throttle_cmd : Outport
  wires:
  FMS_Out/1 -> Bus Selector/1, Error/1(FMS_Out)
  INS_Out/1 -> Error/2(INS_Out), Boosted_Throttle/2(INS_Out)
  Boosted_Throttle/1(boosted_thrust) -> Saturation/1  "boosted_thrust"
  Error/1(vu_cmd_C_mPs) -> PID_Controller/1(vu_cmd_C_mPs)
  PID_Controller/1(thrust_cmd) -> Boosted_Throttle/1(thrust_cmd)
  factor_mc/1 -> Multiply/2, Relay/1
  Logical Operator/1 -> PID_Controller/2(reset)
  Bus Selector/1 -> Logical Operator/1  "<reset>"
  Relay/1 -> Logical Operator/2
  hover_throttle/1 -> Sum1/2
  Saturation/1 -> Sum1/1
  Sum1/1 -> Multiply/1
  Multiply/1 -> throttle_cmd/1

== system Copy_of_Controller/Controller/FW_Controller/Effective_Factor/Fly_Speed/Fly_Direction ==
  INS_Out : Inport
  Bus Selector2 : BusSelector  OutputSignals=vn,ve,vd
  Bus Selector3 : BusSelector  OutputSignals=quat
  Multiply : Product  Multiplication=Matrix(*)
  Mux : Mux  Inputs=3
  Quaternion To DCM : FMT_Model_Lib/Quaternion/Quaternion To DCM
      settings: SourceProductName=FMT Toolbox
  Selector : Selector  InputPortWidth=3  IndexOptions=Index vector (dialog)  Indices=1  OutputSizes=1
  Sign : Signum
  sign : Outport
  wires:
  Bus Selector3/1 -> Quaternion To DCM/1  "<quat>"
  Multiply/1 -> Selector/1
  INS_Out/1 -> Bus Selector3/1, Bus Selector2/1
  Sign/1 -> sign/1
  Mux/1 -> Multiply/2
  Quaternion To DCM/1 -> Multiply/1
  Bus Selector2/2 -> Mux/2  "<ve>"
  Bus Selector2/1 -> Mux/1  "<vn>"
  Selector/1 -> Sign/1  "Vu"
  Bus Selector2/3 -> Mux/3  "<vd>"

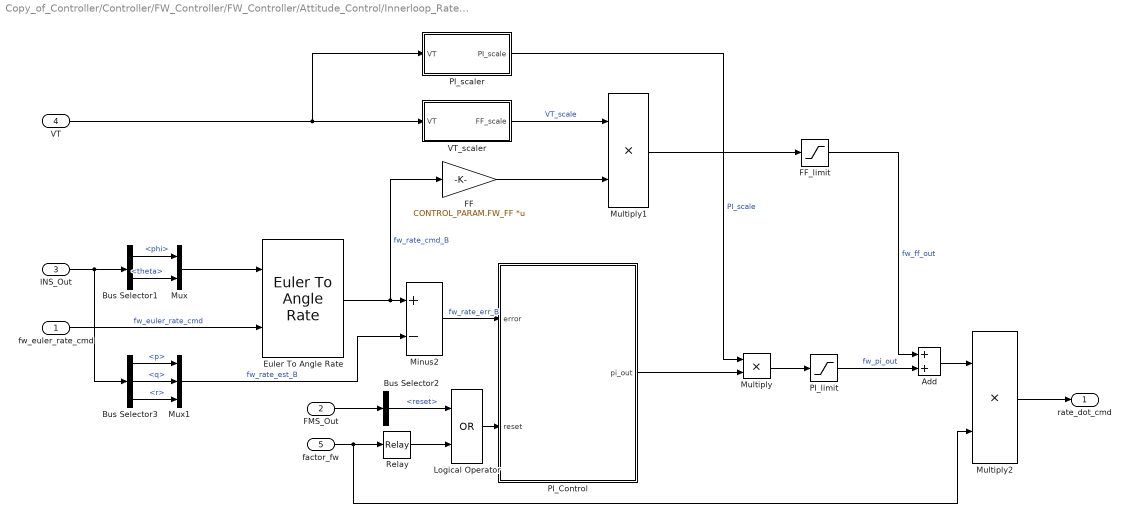
== system Copy_of_Controller/Controller/FW_Controller/FW_Controller/Attitude_Control/Innerloop_Rate_Control ==
  fw_euler_rate_cmd : Inport
  FMS_Out : Inport  Port=2
  INS_Out : Inport  Port=3
  VT : Inport  Port=4
  factor_fw : Inport  Port=5
  Add : Sum
  Bus Selector1 : BusSelector  OutputSignals=phi,theta
  Bus Selector2 : BusSelector  OutputSignals=reset
  Bus Selector3 : BusSelector  OutputSignals=p,q,r
  Euler To Angle Rate : FMT_Model_Lib/Math/Euler To Angle Rate
      settings: SourceProductName=FMT Toolbox
  FF : Gain  Gain=CONTROL_PARAM.FW_FF  Multiplication=Matrix(K*u)
  FF_limit : Saturate  UpperLimit=0.3  LowerLimit=-0.3  OutDataTypeStr=single
  Logical Operator : Logic  Operator=OR  AllPortsSameDT=off  OutDataTypeStr=boolean
  Minus2 : Sum  Inputs=+-
  Multiply : Product
  Multiply1 : Product
  Multiply2 : Product
  Mux : Mux  Inputs=2
  Mux1 : Mux  Inputs=3
  PI_Control : Subsystem
  PI_limit : Saturate  UpperLimit=1  LowerLimit=-1
  PI_scaler : Subsystem
  Relay : Relay  OnSwitchValue=0.3  OffSwitchValue=0.1  OnOutputValue=0  OffOutputValue=1
  VT_scaler : Subsystem
  rate_dot_cmd : Outport
  wires:
  PI_scaler/1(PI_scale) -> Multiply/1  "PI_scale"
  Multiply1/1 -> FF_limit/1
  FF/1 -> Multiply1/2
  FF_limit/1 -> Add/1  "fw_ff_out"
  VT_scaler/1(FF_scale) -> Multiply1/1  "VT_scale"
  fw_euler_rate_cmd/1 -> Euler To Angle Rate/2  "fw_euler_rate_cmd"
  Multiply/1 -> PI_limit/1
  Euler To Angle Rate/1 -> FF/1, Minus2/1  "fw_rate_cmd_B"
  Mux1/1 -> Minus2/2  "fw_rate_est_B"
  PI_limit/1 -> Add/2  "fw_pi_out"
  Add/1 -> Multiply2/1
  Minus2/1 -> PI_Control/1(error)  "fw_rate_err_B"
  Bus Selector2/1 -> Logical Operator/1  "<reset>"
  PI_Control/1(pi_out) -> Multiply/2
  INS_Out/1 -> Bus Selector3/1, Bus Selector1/1
  Bus Selector1/1 -> Mux/1  "<phi>"
  Bus Selector1/2 -> Mux/2  "<theta>"
  Mux/1 -> Euler To Angle Rate/1
  FMS_Out/1 -> Bus Selector2/1
  Bus Selector3/1 -> Mux1/1  "<p>"
  Bus Selector3/2 -> Mux1/2  "<q>"
  Bus Selector3/3 -> Mux1/3  "<r>"
  VT/1 -> PI_scaler/1(VT), VT_scaler/1(VT)
  factor_fw/1 -> Multiply2/2, Relay/1
  Logical Operator/1 -> PI_Control/2(reset)
  Relay/1 -> Logical Operator/2
  Multiply2/1 -> rate_dot_cmd/1

== system Copy_of_Controller/Controller/FW_Controller/FW_Controller/Attitude_Control/Outloop_Angle_Control ==
  att_cmd : Inport
  VT : Inport  Port=2
  INS_Out : Inport  Port=3
  FMS_Out : Inport  Port=4
  Attitude_Controller : Subsystem
  Heading_Controller : Subsystem
  Mux : Mux  Inputs=2
  Reshape : Reshape  OutputDimensionality=Column vector (2-D)
  Signal_Select : Subsystem
  fw_att_cmd : Outport
  fw_euler_rate_cmd : Outport  Port=2
  wires:
  FMS_Out/1 -> Heading_Controller/2(FMS_Out), Signal_Select/2(FMS_Out)
  INS_Out/1 -> Attitude_Controller/2(INS_Out)
  att_cmd/1 -> Signal_Select/1(att_cmd_rad)
  Signal_Select/1(fw_att_cmd) -> Heading_Controller/1(fw_att_cmd), fw_att_cmd/1, Attitude_Controller/1(att_cmd)
  Attitude_Controller/1(phi_theta_rate_cmd) -> Mux/1
  Heading_Controller/1(psi_rate_cmd) -> Mux/2
  Mux/1 -> Reshape/1
  Reshape/1 -> fw_euler_rate_cmd/1
  VT/1 -> Heading_Controller/3(VT)

== system Copy_of_Controller/Controller/FW_Controller/FW_Controller/TECS_Core/path_angle_control ==
  FMS_Out : Inport
  INS_out : Inport  Port=2
  Flight_Path_Angle : Subsystem
  Subsystem : Subsystem
  Sum : Sum  Inputs=|+-
  Target_Flight_Path_Angle : Subsystem
  gamma_err : Outport
  gamma : Outport  Port=2
  wires:
  INS_out/1 -> Flight_Path_Angle/1(INS_Out), Target_Flight_Path_Angle/2(INS_Out), Subsystem/1(INS_Out)
  FMS_Out/1 -> Target_Flight_Path_Angle/1(FMS_Out)
  Target_Flight_Path_Angle/1(gamma_sp) -> Sum/1  "gamma_sp"
  Flight_Path_Angle/1(gamma) -> Sum/2, gamma/1  "gamma"
  Sum/1 -> gamma_err/1
  Subsystem/1(gamma_dir) -> Target_Flight_Path_Angle/3(gamma_dir), Flight_Path_Angle/2(gamma_dir)

== system Copy_of_Controller/Controller/FW_Controller/FW_Controller/TECS_Core/pitch_pid_out ==
  reset : Inport
  B_err : Inport  Port=2
  Add : Sum  Inputs=+++
  D_control : Subsystem
  I_control : Subsystem
  P_control : Gain  Gain=CONTROL_PARAM.FW_TECS_PITCH_P
  Saturation1 : Saturate  UpperLimit=0.3  LowerLimit=-0.3
  pid_out : Outport
  wires:
  B_err/1 -> P_control/1, D_control/1(err), I_control/1(err)
  reset/1 -> I_control/2(reset), D_control/2(reset)
  Add/1 -> pid_out/1
  D_control/1(d_out) -> Saturation1/1
  P_control/1 -> Add/1  "pitch_pout"
  Saturation1/1 -> Add/3  "pitch_dout"
  I_control/1(i_out) -> Add/2  "pitch_iout"

== system Copy_of_Controller/Controller/FW_Controller/FW_Controller/TECS_Core/thorttle_pid_out ==
  E_err : Inport
  reset : Inport  Port=2
  Add4 : Sum  Inputs=+++
  D_control : Subsystem
  I_control : Subsystem
  P_control : Gain  Gain=CONTROL_PARAM.FW_TECS_THOR_P
  Saturation1 : Saturate  UpperLimit=0.3  LowerLimit=-0.3
  pid_out : Outport
  wires:
  E_err/1 -> P_control/1, D_control/1(err), I_control/1(E_err)
  Add4/1 -> pid_out/1
  reset/1 -> I_control/2(reset), D_control/2(reset)
  D_control/1(D_out) -> Saturation1/1
  P_control/1 -> Add4/1  "th_pout"
  I_control/1(i_out) -> Add4/2  "th_iout"
  Saturation1/1 -> Add4/3  "th_dout"

== system Copy_of_Controller/Controller/FW_Controller/FW_Controller/TECS_Core/velocity_control ==
  note: It may not very correct to use ax as Vdot, but diffirence is not too big
  FMS_Out : Inport
  INS_Out : Inport  Port=2
  VT : Inport  Port=3
  Bus Selector : BusSelector  OutputSignals=u_cmd
  Bus Selector2 : BusSelector  OutputSignals=ax
  First Order LPF : FMT_Model_Lib/Filter/First Order LPF  fc=5
      settings: SourceProductName=FMT Toolbox
  Gain : Gain  Gain=1/9.81
  Gain1 : Gain  Gain=1/9.81
  Kv : Gain  Gain=CONTROL_PARAM.FW_TECS_VEL_P
  Minus : Sum  Inputs=+-
  Sum : Sum  Inputs=|+-
  VdotPg : Outport
  VdotPg_err : Outport  Port=2
  wires:
  FMS_Out/1 -> Bus Selector/1
  Gain1/1 -> Sum/2, VdotPg/1  "VdotPg"
  Bus Selector/1 -> Minus/1  "<u_cmd>"
  Gain/1 -> Sum/1  "VdotPg_sp"
  Minus/1 -> Kv/1
  Sum/1 -> VdotPg_err/1  "VdotPg_err"
  VT/1 -> Minus/2
  Bus Selector2/1 -> First Order LPF/1  "<ax>"
  INS_Out/1 -> Bus Selector2/1
  First Order LPF/1 -> Gain1/1
  Kv/1 -> Gain/1

== system Copy_of_Controller/Controller/MC_Controller/Horizontal_Control/Attitude_Controller/Inner_Loop ==
  euler_rate_cmd_radPs : Inport
  INS_Out : Inport  Port=2
  FMS_Out : Inport  Port=3
  Bus Selector : BusSelector  OutputSignals=reset
  Rate_Controller : Subsystem
  Signal_Convert : Subsystem
  Signal_Select : Subsystem
  rate_dot_cmd_B : Outport
  wires:
  euler_rate_cmd_radPs/1 -> Signal_Convert/2(euler_rate_cmd)
  Signal_Select/1(out) -> Rate_Controller/1(rate_cmd_radPs)
  Rate_Controller/1(rate_dot_cmd_B) -> rate_dot_cmd_B/1
  Bus Selector/1 -> Rate_Controller/3(reset)  "<reset>"
  INS_Out/1 -> Signal_Convert/3(INS_Out), Rate_Controller/2(INS_Out)
  FMS_Out/1 -> Signal_Convert/1(FMS_Out), Bus Selector/1, Signal_Select/1(FMS_Out)
  Signal_Convert/1(rate_cmd_radPs) -> Signal_Select/2(rate_cmd_radPs)

== system Copy_of_Controller/Controller/MC_Controller/Horizontal_Control/Attitude_Controller/Outter_Loop ==
  att_cmd_rad : Inport
  INS_Out : Inport  Port=2
  FMS_Out : Inport  Port=3
  Attitude_Controller : Subsystem
  Signal_Select : Subsystem
  euler_rate_cmd_radPs : Outport
  wires:
  Signal_Select/1(out) -> Attitude_Controller/1(att_cmd_rad)
  FMS_Out/1 -> Signal_Select/2(FMS_Out)
  INS_Out/1 -> Attitude_Controller/2(INS_Out)
  Attitude_Controller/1(euler_rate_cmd_radPs) -> euler_rate_cmd_radPs/1
  att_cmd_rad/1 -> Signal_Select/1(att_cmd_rad)

== system Copy_of_Controller/Controller/MC_Controller/Horizontal_Control/Velocity_Controller/Accel_to_Attitude_CMD ==
  note: Gain to resist
      | air drag
  accel_cmd_C_mPs2 : Inport
  Atan : Trigonometry  Operator=atan
  Divide : Product  Inputs=*/
  Gain1 : Gain  Gain=-1
  Mux : Mux  Inputs=2
  Saturation : Saturate  UpperLimit=CONTROL_PARAM.MC_ROLL_PITCH_CMD_LIM  LowerLimit=-CONTROL_PARAM.MC_ROLL_PITCH_CMD_LIM
  Selector : Selector  InputPortWidth=2  IndexOptions=Index vector (dialog)  Indices=1  OutputSizes=1
  Selector1 : Selector  InputPortWidth=2  IndexOptions=Index vector (dialog)  Indices=2  OutputSizes=1
  g : Constant  Value=9.8055  OutDataTypeStr=single
  gain : Gain  Gain=1.1
  att_cmd_B_rad : Outport
  wires:
  Mux/1 -> gain/1
  gain/1 -> Divide/1
  Atan/1 -> Saturation/1
  g/1 -> Divide/2
  Divide/1 -> Atan/1
  Selector/1 -> Gain1/1
  Selector1/1 -> Mux/1
  accel_cmd_C_mPs2/1 -> Selector/1, Selector1/1
  Gain1/1 -> Mux/2
  Saturation/1 -> att_cmd_B_rad/1

== system Copy_of_Controller/Controller/MC_Controller/Horizontal_Control/Velocity_Controller/Error ==
  INS_Out : Inport
  FMS_Out : Inport  Port=2
  Bus Selector : BusSelector  OutputSignals=u_cmd,v_cmd
  Bus_Select : Subsystem
  Mux : Mux  Inputs=2
  Sum : Sum  Inputs=|+-
  TD : Subsystem
  uv_err_C_mPs : Outport
  wires:
  Sum/1 -> uv_err_C_mPs/1  "uv_error_C_mPs"
  FMS_Out/1 -> Bus Selector/1
  INS_Out/1 -> Bus_Select/1(INS_Out)
  Bus Selector/1 -> Mux/1  "<u_cmd>"
  Bus Selector/2 -> Mux/2  "<v_cmd>"
  Mux/1 -> TD/1(v)
  Bus_Select/1(uv_est_C_mPs) -> Sum/2  "uv_est_C_mPs"
  TD/1(v1) -> Sum/1  "uv_cmd_C_mPs"

== system Copy_of_Controller/Controller/MC_Controller/Horizontal_Control/Velocity_Controller/PID_Controller ==
  uv_err_C_mPs : Inport
  reset : Inport  Port=2
  Add : Sum  Inputs=+++
  D_Control : Subsystem  mask{kd=CONTROL_PARAM.MC_VEL_XY_D, max_d=CONTROL_PARAM.MC_VEL_XY_D_MAX, min_d=CONTROL_PARAM.MC_VEL_XY_D_MIN}
  I_Control : Subsystem  mask{ki=CONTROL_PARAM.MC_VEL_XY_I, max_i=CONTROL_PARAM.MC_VEL_XY_I_MAX, min_i=CONTROL_PARAM.MC_VEL_XY_I_MIN}
  P_Control : Subsystem  mask{kp=CONTROL_PARAM.MC_VEL_XY_P}
  accel_cmd_C : Outport
  wires:
  uv_err_C_mPs/1 -> P_Control/1(err), I_Control/1(err), D_Control/1(err)
  reset/1 -> I_Control/2(reset), D_Control/2(reset)
  P_Control/1(p_out) -> Add/1  "accel_p_out"
  I_Control/1(i_out) -> Add/2  "accel_i_out"
  D_Control/1(d_out) -> Add/3  "accel_d_out"
  Add/1 -> accel_cmd_C/1

== system Copy_of_Controller/Controller/MC_Controller/Horizontal_Control/Velocity_Controller/Signal_Select ==
  acc_cmd_in : Inport
  FMS_Out : Inport  Port=2
  Bus Selector : BusSelector  OutputSignals=ctrl_mode
  Offboard : simulink/Logic and Bit Operations/Compare To Constant  relop===  const=uint8(ControlMode.Offboard)  OutDataTypeStr=boolean
  Offboard_Signal_Select : Subsystem
  Switch : Switch  Criteria=u2 > Threshold
  acc_cmd_out : Outport
  wires:
  FMS_Out/1 -> Offboard_Signal_Select/1(FMS_Out), Bus Selector/1
  Bus Selector/1 -> Offboard/1  "<ctrl_mode>"
  Offboard/1 -> Switch/2
  Switch/1 -> acc_cmd_out/1
  acc_cmd_in/1 -> Offboard_Signal_Select/2(acc_cmd_in), Switch/3
  Offboard_Signal_Select/1(acc_cmd) -> Switch/1

== system Copy_of_Controller/Controller/MC_Controller/Vertical_Control/Veloxity_Z_Controller/Boosted_Throttle ==
  thrust_cmd : Inport
  INS_Out : Inport  Port=2
  Bus Selector : BusSelector  OutputSignals=phi,theta
  Constant : Constant  OutDataTypeStr=single
  Cos : Trigonometry  Operator=cos
  Cos1 : Trigonometry  Operator=cos
  Divide : Product  Inputs=*/
  Gain : Gain  Gain=2
  Multiply : Product
  Multiply1 : Product  Inputs=3
  Saturation : Saturate  UpperLimit=1  LowerLimit=0
  Saturation1 : Saturate  UpperLimit=1  LowerLimit=0.5
  boosted_thrust : Outport
  wires:
  INS_Out/1 -> Bus Selector/1
  Bus Selector/1 -> Cos/1  "<phi>"
  Bus Selector/2 -> Cos1/1  "<theta>"
  Cos/1 -> Multiply/1
  Cos1/1 -> Multiply/2
  Multiply/1 -> Saturation1/1, Gain/1
  Gain/1 -> Saturation/1
  Saturation/1 -> Multiply1/3  "inverted_factor"
  Constant/1 -> Divide/1
  Divide/1 -> Multiply1/2  "boost_factor"
  Saturation1/1 -> Divide/2
  thrust_cmd/1 -> Multiply1/1
  Multiply1/1 -> boosted_thrust/1

== system Copy_of_Controller/Controller/MC_Controller/Vertical_Control/Veloxity_Z_Controller/Error ==
  FMS_Out : Inport
  INS_Out : Inport  Port=2
  Bus Selector1 : BusSelector  OutputSignals=vd
  Bus Selector2 : BusSelector  OutputSignals=w_cmd
  Gain : Gain  Gain=-1  OutDataTypeStr=Inherit: Same as input
  Signal Copy1 : SignalConversion  OverrideOpt=off
  Sum1 : Sum  Inputs=|+-
  TD : Subsystem
  vu_cmd_C_mPs : Outport
  wires:
  INS_Out/1 -> Bus Selector1/1
  Bus Selector2/1 -> TD/1(v)  "<w_cmd>"
  Bus Selector1/1 -> Signal Copy1/1  "<vd>"
  Gain/1 -> vu_cmd_C_mPs/1
  Sum1/1 -> Gain/1  "w_error_C_mPs"
  FMS_Out/1 -> Bus Selector2/1
  TD/1(v1) -> Sum1/1  "w_cmd_C_mPs"
  Signal Copy1/1 -> Sum1/2  "w_est_C_mPs"

== system Copy_of_Controller/Controller/MC_Controller/Vertical_Control/Veloxity_Z_Controller/PID_Controller ==
  vu_cmd_C_mPs : Inport
  reset : Inport  Port=2
  Add : Sum  Inputs=+++
  D_Control : Subsystem  mask{kd=CONTROL_PARAM.MC_VEL_Z_D, max_d=CONTROL_PARAM.MC_VEL_Z_D_MAX, min_d=CONTROL_PARAM.MC_VEL_Z_D_MIN}
  I_Control : Subsystem  mask{ki=CONTROL_PARAM.MC_VEL_Z_I, max_i=CONTROL_PARAM.MC_VEL_Z_I_MAX, min_i=CONTROL_PARAM.MC_VEL_Z_I_MIN}
  P_Control : Subsystem  mask{kp=CONTROL_PARAM.MC_VEL_Z_P}
  thrust_cmd : Outport
  wires:
  P_Control/1(p_out) -> Add/1  "thrust_p_out"
  I_Control/1(i_out) -> Add/2  "thrust_i_out"
  Add/1 -> thrust_cmd/1
  vu_cmd_C_mPs/1 -> D_Control/1(err), I_Control/1(err), P_Control/1(err)
  D_Control/1(d_out) -> Add/3  "thrust_d_out"
  reset/1 -> I_Control/2(reset), D_Control/2(reset)
